simulink model "correctionrs_test"  (R2020b)
settings: Solver=VariableStepAuto  StartTime=0.0  StopTime=10.0  RelTol=1e-3
settings Model: Creator=Dona  LastModifiedBy=Dona

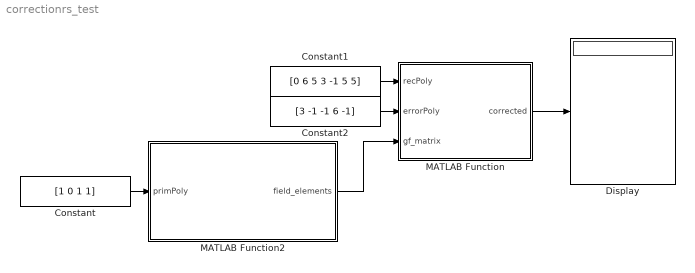
== system correctionrs_test ==
  Constant : Constant  Value=[1 0 1 1]
  Constant1 : Constant  Value=[0 6 5 3 -1 5 5]  VectorParams1D=off
  Constant2 : Constant  Value=[3 -1 -1 6 -1]  VectorParams1D=off
  Display : Display
  MATLAB Function : MATLAB Function  TreatAsAtomicUnit=on
  MATLAB Function2 : MATLAB Function  TreatAsAtomicUnit=on
  wires:
  MATLAB Function/1(corrected) -> Display/1
  Constant/1 -> MATLAB Function2/1(primPoly)
  MATLAB Function2/1(field_elements) -> MATLAB Function/3(gf_matrix)
  Constant1/1 -> MATLAB Function/1(recPoly)
  Constant2/1 -> MATLAB Function/2(errorPoly)

== matlab function correctionrs_test/MATLAB Function2 ==
  data: primPoly input; field_elements output
% GenerateGF2m: generates the selected Galois Field element. The inputs should be the
% order m and the coefficients of an appropriate primitive polynomial. The generated field,
% in either binary or power notation, may be a calling parameter for each of the other
% functions. Hint: I strongly suggest that you input the coefficients in “power” notation,
% with the highest order power on the left

function field_elements  = GenerateGF2m(primPoly) %primPoly in power notation, highest order on left

m = 3;
% hard coded size of retrun matrices and gf mtrix because simulink
% whines about variable output size. Havent figured out how to fix it
% ask laberge
gf = zeros(8, 3); %there are 2^m field elements
field_elements = zeros(8, 3); %there are 2^m field elements

gfIndx = 2; %gfIndx(1) holds initial state 
numShifts = (2^m) - 1;
s_reg = zeros(1,int8(m));
s_reg(end) = 1; %rightmost element of init shr is 1
gf(1, :) = 0;%write the contents of the init shift register to the matrix of gf elements
gf(2, :) = s_reg;
for i = 2:numShifts %number of shifts corresponds to power of primitive element
    carryOut = s_reg(1);%save the value to be wrapped
    for i0 = 1:numel(s_reg)-1
        if primPoly(i0 + 1) == 1
            s_reg(i0) = xor(carryOut, s_reg(i0 + 1));
        else
            s_reg(i0) = s_reg(i0 + 1);
        end
    end
    s_reg(end) = carryOut;
    gf(i+1,:) = s_reg; %add the newly shifted register to the gf matrix
end
field_elements = gf;
end

== matlab function correctionrs_test/MATLAB Function ==
  data: recPoly input; corrected output; errorPoly input; gf_matrix input
function corrected  = CorrectionRS(recPoly,errorPoly, gf_matrix)

%pad the error polynomial with inf if necessary
errorExp = -1*ones(1, numel(recPoly));
errorExp_i = numel(errorExp);
for j = numel(errorPoly):-1:1
    errorExp(errorExp_i) = errorPoly(j);
    errorExp_i = errorExp_i - 1;
end

%This function corrects a codeword polynomial given the error polynomial
corrected = -1*ones(1, numel(recPoly));
for i = 1: numel(corrected)
    corrected(i) = AddGF2m(recPoly(i), errorExp(i), gf_matrix);
end
%    printres = ['The corrected word is: ', num2str(corrected(:).'), '. Decoding complete.'];
%    disp(printres);
%end
